simulink model "shellModels"  (R2023b)
settings: Solver=VariableStepAuto  StartTime=0.0  StopTime=10.0  RelTol=1e-3
undefined symbols (not defined in the file or in its folder): inertia, mass
settings Model: Creator=sgopalswamy  LastModifiedBy=sgopalswamy

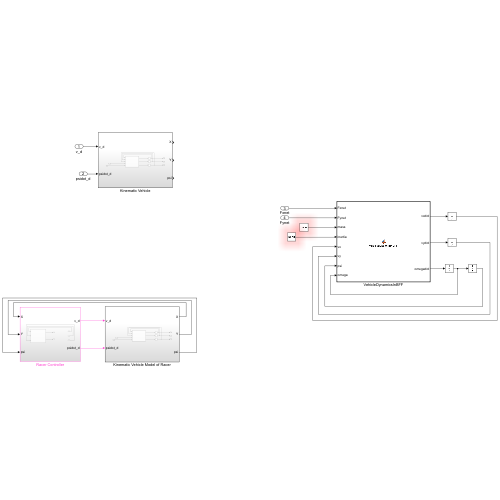
[thumbnail: Simulink's stored preview of the top-level diagram]
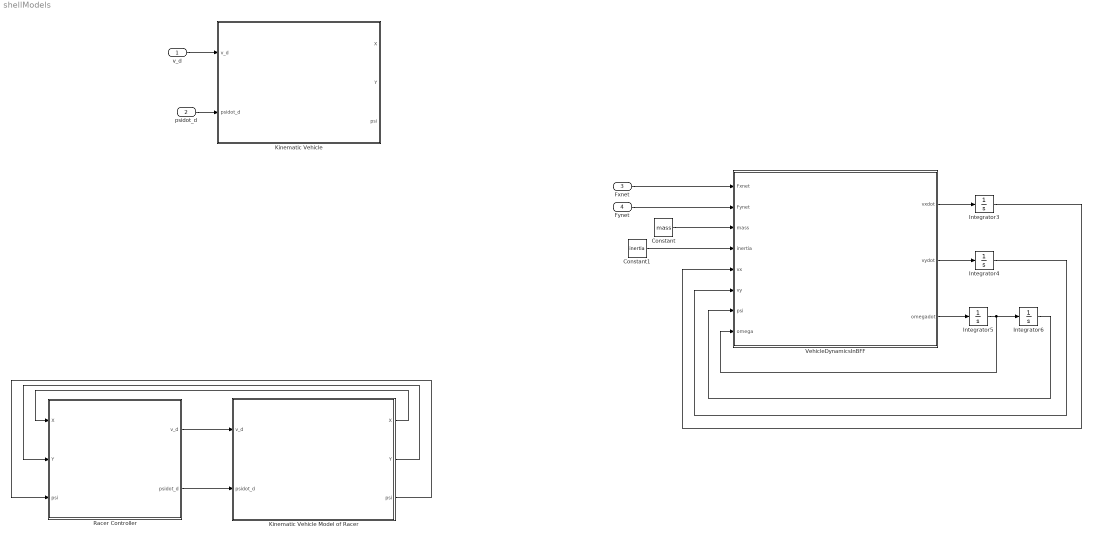
== system shellModels ==
  v_d : Inport
  psidot_d : Inport  Port=2
  Fxnet : Inport  Port=3
  Fynet : Inport  Port=4
  Constant : Constant  Value=mass
  Constant1 : Constant  Value=inertia
  Integrator{3..6} (4 alike) : Integrator
  Kinematic Vehicle : Subsystem
  Kinematic Vehicle Model of Racer : Subsystem
  Racer Controller : Subsystem
  VehicleDynamicsInBFF : MATLAB Function  TreatAsAtomicUnit=on
  wires:
  VehicleDynamicsInBFF/1(vxdot) -> Integrator3/1
  VehicleDynamicsInBFF/2(vydot) -> Integrator4/1
  VehicleDynamicsInBFF/3(omegadot) -> Integrator5/1
  Integrator5/1 -> VehicleDynamicsInBFF/8(omega), Integrator6/1
  Integrator6/1 -> VehicleDynamicsInBFF/7(psi)
  Integrator4/1 -> VehicleDynamicsInBFF/6(vy)
  Integrator3/1 -> VehicleDynamicsInBFF/5(vx)
  Fxnet/1 -> VehicleDynamicsInBFF/1(Fxnet)
  Fynet/1 -> VehicleDynamicsInBFF/2(Fynet)
  Constant/1 -> VehicleDynamicsInBFF/3(mass)
  Constant1/1 -> VehicleDynamicsInBFF/4(inertia)
  v_d/1 -> Kinematic Vehicle/1(v_d)
  psidot_d/1 -> Kinematic Vehicle/2(psidot_d)
  Kinematic Vehicle Model of Racer/1(X) -> Racer Controller/1(X)
  Kinematic Vehicle Model of Racer/2(Y) -> Racer Controller/2(Y)
  Kinematic Vehicle Model of Racer/3(psi) -> Racer Controller/3(psi)
  Racer Controller/1(v_d) -> Kinematic Vehicle Model of Racer/1(v_d)
  Racer Controller/2(psidot_d) -> Kinematic Vehicle Model of Racer/2(psidot_d)

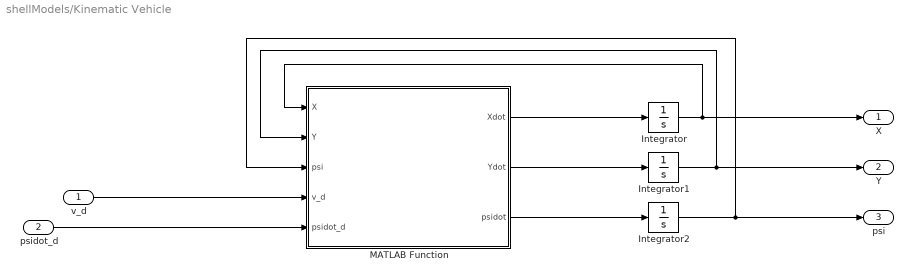
== system shellModels/Kinematic Vehicle ==
  v_d : Inport
  psidot_d : Inport  Port=2
  Integrator : Integrator
  Integrator1 : Integrator
  Integrator2 : Integrator
  MATLAB Function : MATLAB Function  TreatAsAtomicUnit=on
  X : Outport
  Y : Outport  Port=2
  psi : Outport  Port=3
  wires:
  Integrator1/1 -> Y/1, MATLAB Function/2(Y)
  Integrator2/1 -> psi/1, MATLAB Function/3(psi)
  Integrator/1 -> MATLAB Function/1(X), X/1
  MATLAB Function/3(psidot) -> Integrator2/1
  MATLAB Function/2(Ydot) -> Integrator1/1
  psidot_d/1 -> MATLAB Function/5(psidot_d)
  MATLAB Function/1(Xdot) -> Integrator/1
  v_d/1 -> MATLAB Function/4(v_d)

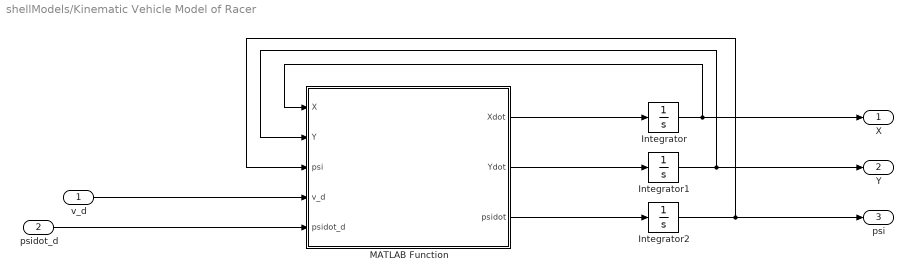
== system shellModels/Kinematic Vehicle Model of Racer ==
  v_d : Inport
  psidot_d : Inport  Port=2
  Integrator : Integrator
  Integrator1 : Integrator
  Integrator2 : Integrator
  MATLAB Function : MATLAB Function  TreatAsAtomicUnit=on
  X : Outport
  Y : Outport  Port=2
  psi : Outport  Port=3
  wires:
  v_d/1 -> MATLAB Function/4(v_d)
  MATLAB Function/1(Xdot) -> Integrator/1
  psidot_d/1 -> MATLAB Function/5(psidot_d)
  MATLAB Function/2(Ydot) -> Integrator1/1
  MATLAB Function/3(psidot) -> Integrator2/1
  Integrator/1 -> X/1, MATLAB Function/1(X)
  Integrator2/1 -> MATLAB Function/3(psi), psi/1
  Integrator1/1 -> MATLAB Function/2(Y), Y/1

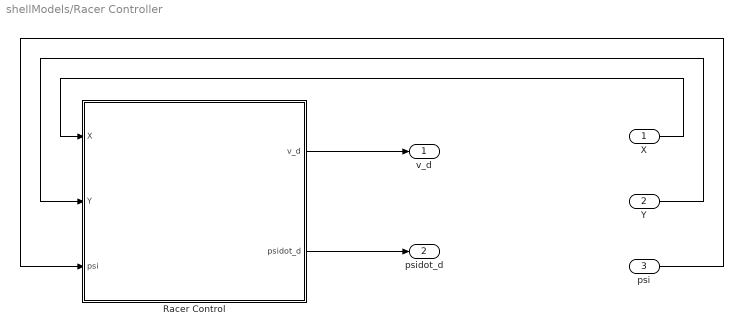
== system shellModels/Racer Controller ==
  X : Inport
  Y : Inport  Port=2
  psi : Inport  Port=3
  Racer Control : MATLAB Function  TreatAsAtomicUnit=on
  v_d : Outport
  psidot_d : Outport  Port=2
  wires:
  Racer Control/2(psidot_d) -> psidot_d/1
  psi/1 -> Racer Control/3(psi)
  X/1 -> Racer Control/1(X)
  Y/1 -> Racer Control/2(Y)
  Racer Control/1(v_d) -> v_d/1

== matlab function shellModels/VehicleDynamicsInBFF ==
  data: Fxnet input; vxdot output; Fynet input; mass input; inertia input; vx input; vy input; psi input; omega input; vydot output; omegadot output
function [vxdot, vydot, omegadot] = VehicleDynamicsInBFF(Fxnet, Fynet, mass, inertia, vx, vy, psi, omega)

y = u;

== matlab function shellModels/Kinematic Vehicle/MATLAB Function ==
  data: X input; Xdot output; Y input; psi input; v_d input; psidot_d input; Ydot output; psidot output
function [Xdot, Ydot, psidot] = kinematicVehicle(X, Y, psi, v_d, psidot_d)

y = u;

== matlab function shellModels/Kinematic Vehicle Model of Racer/MATLAB Function ==
  data: X input; Xdot output; Y input; psi input; v_d input; psidot_d input; Ydot output; psidot output
function [Xdot, Ydot, psidot] = kinematicVehicle(X, Y, psi, v_d, psidot_d)

y = u;

== matlab function shellModels/Racer Controller/Racer Control ==
  data: X input; v_d output; Y input; psi input; psidot_d output
function [v_d, psidot_d] = fcn(X,Y,psi)

y = u;
